simulink model "LAB4_Simulink"  (R2024b)
settings: Solver=VariableStepAuto  StartTime=0.0  StopTime=10  MaxStep=1e-3  RelTol=1e-3
values from neighbouring files (symbols this model uses):
  A = [0 1; 2*Km*Im^2/(m*x1_eq^3) 0]    [LAB4_Levitator_parameter_and_design.m]
  alfa = inv(-(C-D*K)*inv(A-B*K)*B + D)    [LAB4_Levitator_parameter_and_design.m]
  B = [0; -2*Km*Im/(m*x1_eq^2)]    [LAB4_Levitator_parameter_and_design.m]
  C = [Kt 0]    [LAB4_Levitator_parameter_and_design.m]
  g = 9.81    [LAB4_Levitator_parameter_and_design.m]
  Im = 0.8    [LAB4_Levitator_parameter_and_design.m]
  K = place(A,B,p_k)    [LAB4_Levitator_parameter_and_design.m]
  Km = 1.52e-4    (= 0.000152)    [LAB4_Levitator_parameter_and_design.m]
  Kt = 708.27    [LAB4_Levitator_parameter_and_design.m]
  L = place(A',C',p_l)'    [LAB4_Levitator_parameter_and_design.m]
  m = 0.02    [LAB4_Levitator_parameter_and_design.m]
  x1_eq = Im*sqrt(Km/(m*g))    [LAB4_Levitator_parameter_and_design.m]
settings Model: Creator=cristiansapia  LastModifiedBy=stefa
settings DebuggingCC: UnconnectedInputMsg=warning  UnconnectedOutputMsg=warning  UnconnectedLineMsg=warning
settings ModelReferenceCC: EnableRefExpFcnMdlSchedulingChecks=on
settings RTWCC: GPUComputeCapability=3.5  DLArmComputeVersion=19.05

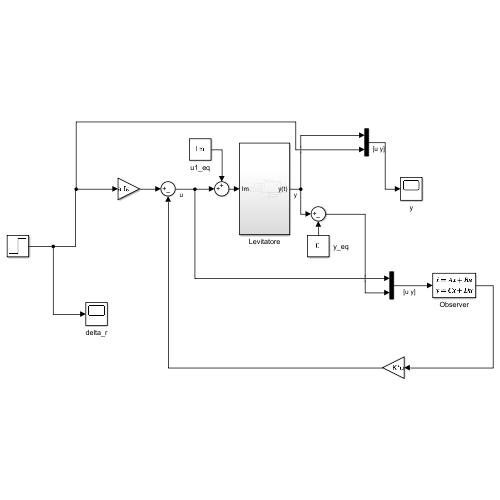
[thumbnail: Simulink's stored preview of the top-level diagram]
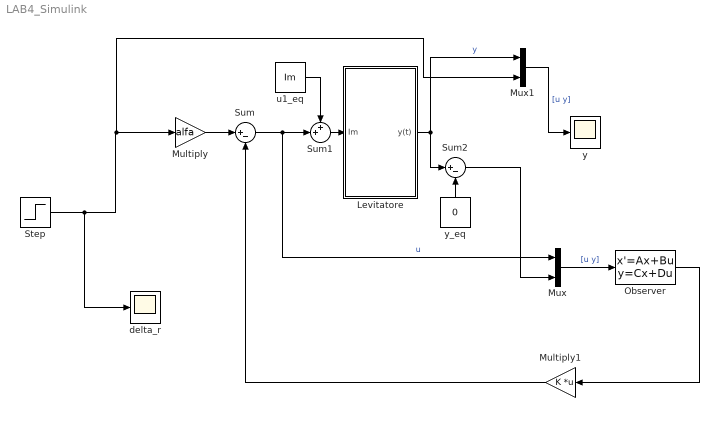
== system LAB4_Simulink ==
  Levitatore : Subsystem
  Multiply : Gain  Gain=alfa
  Multiply1 : Gain  Gain=K  Multiplication=Matrix(K*u)
  Mux : Mux  Inputs=2
  Mux1 : Mux  Inputs=2
  Observer : StateSpace  A=A-L*C  B=[B L]  C=eye(2,2)  D=zeros(2,2)  InitialCondition=0
  Step : Step  Time=0  After=7  SampleTime=0
  Sum : Sum  Inputs=|+-
  Sum1 : Sum  Inputs=++|
  Sum2 : Sum  Inputs=|+-
  delta_r : Scope
  u1_eq : Constant  Value=Im
  y : Scope
  y_eq : Constant  Value=0
  wires:
  Mux/1 -> Observer/1  "[u y]"
  Levitatore/1(y(t)) -> Sum2/1, Mux1/1  "y"
  Multiply1/1 -> Sum/2
  Observer/1 -> Multiply1/1
  Sum1/1 -> Levitatore/1(Im)
  u1_eq/1 -> Sum1/1
  y_eq/1 -> Sum2/2
  Sum2/1 -> Mux/2
  Sum/1 -> Mux/1, Sum1/2  "u"
  Multiply/1 -> Sum/1
  Step/1 -> delta_r/1, Mux1/2, Multiply/1
  Mux1/1 -> y/1  "[u y]"

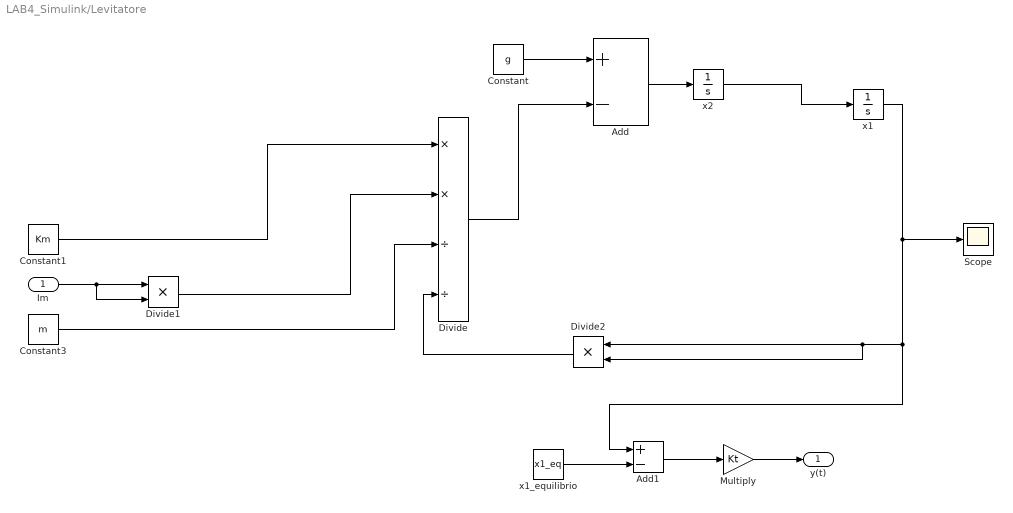
== system LAB4_Simulink/Levitatore ==
  Im : Inport
  Add : Sum  Inputs=+-
  Add1 : Sum  Inputs=+-
  Constant : Constant  Value=g
  Constant1 : Constant  Value=Km
  Constant3 : Constant  Value=m
  Divide : Product  Inputs=**//
  Divide1 : Product  Inputs=**
  Divide2 : Product  Inputs=**
  Multiply : Gain  Gain=Kt
  Scope : Scope
  x1 : Integrator  InitialCondition=x1_eq
  x1_equilibrio : Constant  Value=x1_eq
  x2 : Integrator
  y(t) : Outport
  wires:
  Divide2/1 -> Divide/4
  Constant1/1 -> Divide/1
  Constant3/1 -> Divide/3
  Add/1 -> x2/1
  Constant/1 -> Add/1
  x1/1 -> Scope/1, Add1/1, Divide2/2, Divide2/1
  Divide/1 -> Add/2
  Divide1/1 -> Divide/2
  Im/1 -> Divide1/2, Divide1/1
  x1_equilibrio/1 -> Add1/2
  Add1/1 -> Multiply/1
  Multiply/1 -> y(t)/1
  x2/1 -> x1/1
